simulink model "PV_Model"  (R2025b)
settings: Solver=ode23tb  StartTime=0.0  StopTime=2  MaxStep=1e-4  RelTol=1e-3
libraries: spsCurrentMeasurementLib x1, spsGroundLib x1, spsPVArrayLib x1, spsSeriesRLCBranchLib x1, spsVoltageMeasurementLib x1, spspowerguiLib x1
settings Model: Creator=hp  LastModifiedBy=hp

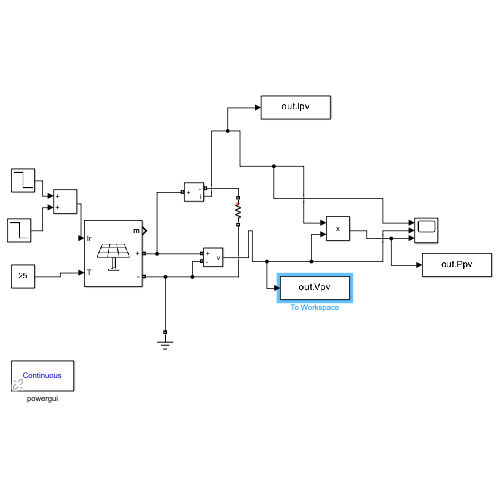
[thumbnail: Simulink's stored preview of the top-level diagram]
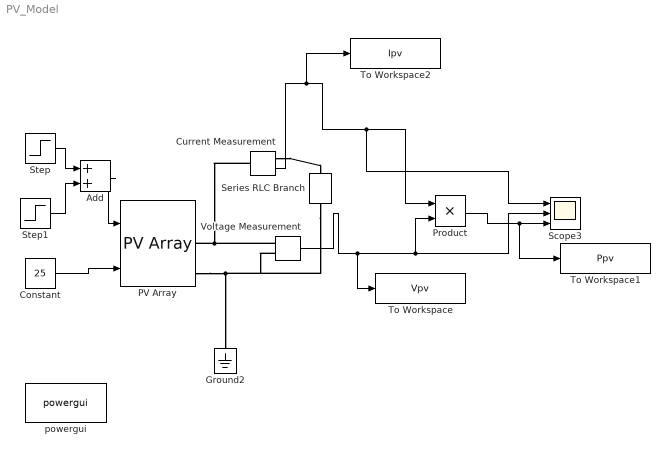
== system PV_Model ==
  Add : Sum
  Constant : Constant  Value=25
  Current Measurement : spsCurrentMeasurementLib/Current Measurement  PhasorSimulation=off  OutputType=Complex  PSBequivalent=0
  Ground2 : spsGroundLib/Ground  LConnTagsString=a
  PV Array : spsPVArrayLib/PV Array  Npar=2  Nser=10  PlotType=array @ 25 deg.C & specified irradiances  S_vec="[ 1000  ]"  Temp_C_vec="[ 45 25  ]"  ModuleName=User-defined  PlotWhenSelected=off  Pm=76.5  Ncell=60  Voc=21  Isc=5  Vm=17  Im=4.5  beta_Voc_pc=-0.36099  alpha_Isc_pc=0.102  beta_Voc=-0.075808  alpha_Isc=0.0051  IL=5.0239  I0=1.8232e-10  nI=0.56827  Rsh=64.5342  Rs=0.30904  RobustModel=off  RobustCellTemperature=313.3991  BAL=on  Tc=1e-6  Tfilter=5e-5
  Product : Product
  Scope3 : Scope  NumInputPorts=3
      settings: ActiveDisplayYMinimum=-1  ActiveDisplayYMaximum=1  DataLoggingVariableName=ScopeData3
  Series RLC Branch : spsSeriesRLCBranchLib/Series RLC Branch  LConnTagsString=__new0  RConnTagsString=__new0  BranchType=R  Resistance=20  Inductance=1e-3  SetiL0=off  InitialCurrent=0  Capacitance=1e-6  Setx0=off  InitialVoltage=0  Measurements=None
  Step : Step  Time=0.5  Before=1000  After=800  SampleTime=0
  Step1 : Step  After=-200  SampleTime=0
  To Workspace : ToWorkspace  VariableName=Vpv  SampleTime=-1
  To Workspace1 : ToWorkspace  VariableName=Ppv  SampleTime=-1
  To Workspace2 : ToWorkspace  VariableName=Ipv  SampleTime=-1
  Voltage Measurement : spsVoltageMeasurementLib/Voltage Measurement  PhasorSimulation=off  OutputType=Complex  PSBequivalent=0
  powergui : spspowerguiLib/powergui  Priority=1  SimulationMode=Continuous  SampleTime=50e-6  frequency=60  Iterations=50  frequencyindice=0  Pbase=100e6  ErrMax=1e-4  UnitsV=kV  UnitsW=MW  buscounter=0  FunctionMessages=off  echomessages=off  EnableUseOfTLC=off  CurrentSourceSwitches=off  DisableSnubberDevices=off  DisableRonSwitches=off  DisableVfSwitches=off  DisplayEquations=off  AutomaticDiscreteSolvers=off  SolverType=Tustin/Backward Euler (TBE)  Interpol=off  ExternalGateDelay=off  methode=off  Ts=100  x0status=blocks  SPID=on  SwTol=0  HookPort=off  NonlinearTolerance=1e-4  nMaxIteration=100  ContinueOnMaxIteration=off  RestoreLinks=warning  ResistiveCurrentMeasurement=off  Frange=[0:2:500]  Ylog=off  Xlog=on  ShowGrid=off  save=off  variable=ZData  structure=0  ZoomFFT=off  StartTime=0.0  cycles=1  DisplayStyle=1  fundamental=60  FreqAxis=off  MaxFrequency=1000  frequencyindicesteady=1  RmsSteady=1  display=off
  wires:
  Voltage Measurement/1 -> To Workspace/1, Scope3/2, Product/2
  Constant/1 -> PV Array/2
  Current Measurement/1 -> To Workspace2/1, Scope3/1, Product/1
  Product/1 -> To Workspace1/1, Scope3/3
  Add/1 -> PV Array/1
  Step/1 -> Add/1
  Step1/1 -> Add/2
  connections:
  PV Array/RConn2 -- Series RLC Branch/RConn1 -- Voltage Measurement/LConn2 -- Ground2/LConn1
  Voltage Measurement/LConn1 -- Current Measurement/LConn1 -- PV Array/RConn1
  Current Measurement/RConn1 -- Series RLC Branch/LConn1
